simulink model "DCMotor_Para_Est_2021b"  (R2021b)
settings: Solver=VariableStepAuto  StartTime=0.0  StopTime=10.0  RelTol=1e-3
libraries: arduinolib x2, arduinosensorlib x1
settings Model: Creator=LabPC  LastModifiedBy=LabPC
settings DebuggingCC: UnconnectedInputMsg=none  UnconnectedOutputMsg=none  UnconnectedLineMsg=none
settings RTWCC: DLArmComputeVersion=20.02.1

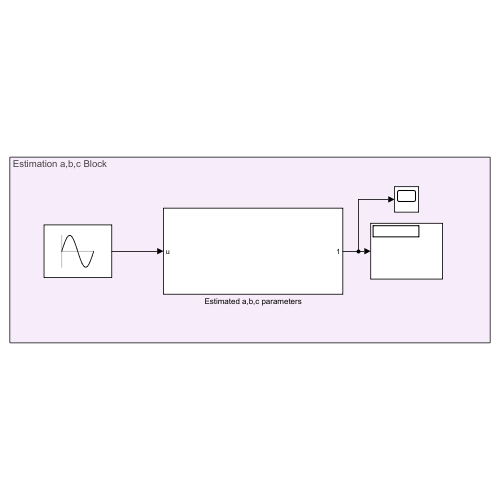
[thumbnail: Simulink's stored preview of the top-level diagram]
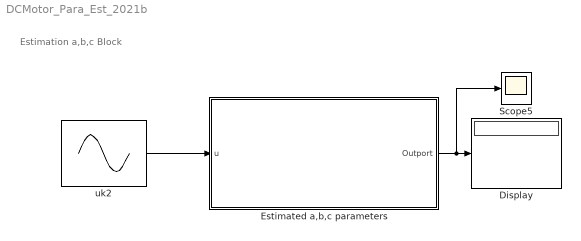
== system DCMotor_Para_Est_2021b ==
  note: Estimation a,b,c Block
  Display : Display
  Estimated a,b,c parameters : Subsystem
  Scope5 : Scope
  uk2 : Sin  Amplitude=12  Frequency=2*pi*1.2  SampleTime=0
  wires:
  Estimated a,b,c parameters/1(Outport) -> Scope5/1, Display/1
  uk2/1 -> Estimated a,b,c parameters/1(u)

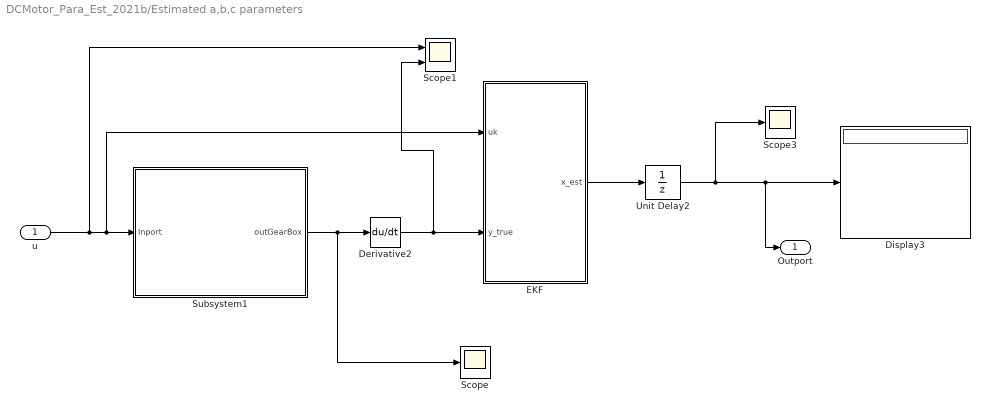
== system DCMotor_Para_Est_2021b/Estimated a,b,c parameters ==
  u : Inport
  Derivative2 : Derivative
  Display3 : Display
  EKF : MATLAB Function  TreatAsAtomicUnit=on
  Scope : Scope
  Scope1 : Scope  NumInputPorts=2
  Scope3 : Scope
  Subsystem1 : Subsystem
  Unit Delay2 : UnitDelay  InitialCondition=[0;0;0;0]  SampleTime=-1  HasFrameUpgradeWarning=on
  Outport : Outport
  wires:
  Derivative2/1 -> Scope1/2, EKF/2(y_true)
  Unit Delay2/1 -> Outport/1, Display3/1, Scope3/1
  EKF/1(x_est) -> Unit Delay2/1
  Subsystem1/1(outGearBox) -> Scope/1, Derivative2/1
  u/1 -> Scope1/1, Subsystem1/1(Inport), EKF/1(uk)

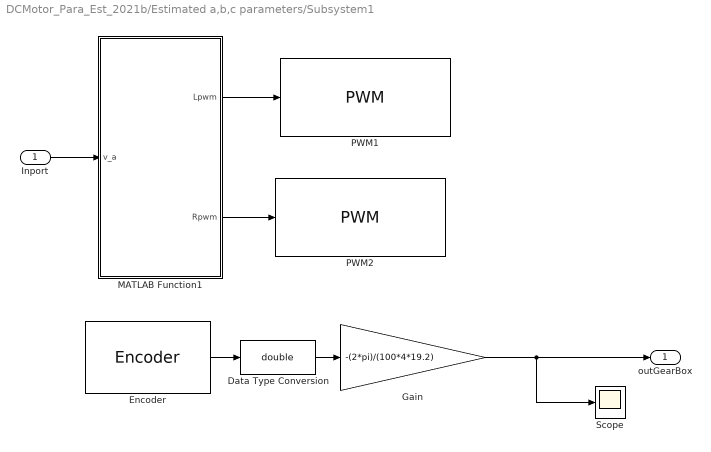
== system DCMotor_Para_Est_2021b/Estimated a,b,c parameters/Subsystem1 ==
  Inport : Inport
  Data Type Conversion : DataTypeConversion  OutDataTypeStr=double
  Encoder : arduinosensorlib/Encoder  InputA=2  InputB=3  Mode=No reset  SampleTime=-1
      settings: SourceProductBaseCode=ARDUINO
  Gain : Gain  Gain=-(2*pi)/(100*4*19.2)
  MATLAB Function1 : MATLAB Function  TreatAsAtomicUnit=on
  PWM1 : arduinolib/PWM  pinNumber=6  frequencyType=Default  desiredFrequency=490.2  achievableFrequency=490.2
  PWM2 : arduinolib/PWM  pinNumber=7  frequencyType=Default  desiredFrequency=490.2  achievableFrequency=490.2
  Scope : Scope
  outGearBox : Outport
  wires:
  Gain/1 -> Scope/1, outGearBox/1
  Encoder/1 -> Data Type Conversion/1
  Data Type Conversion/1 -> Gain/1
  MATLAB Function1/1(Lpwm) -> PWM1/1
  MATLAB Function1/2(Rpwm) -> PWM2/1
  Inport/1 -> MATLAB Function1/1(v_a)

== matlab function DCMotor_Para_Est_2021b/Estimated a,b,c parameters/Subsystem1/MATLAB Function1 ==
  data: v_a input; Lpwm output; Rpwm output
function [Lpwm,Rpwm] = fcn(v_a)

vmax = 22.9;
pwm_cal = v_a*254/vmax;

if pwm_cal > 0
    Lpwm = 0;
    Rpwm = pwm_cal;
elseif pwm_cal < 0
    Lpwm = abs(pwm_cal);
    Rpwm = 0;
else
    Lpwm = 0;
    Rpwm = 0;
end

== matlab function DCMotor_Para_Est_2021b/Estimated a,b,c parameters/EKF ==
  settings: updateMethod=DISCRETE
  data: uk input; y_true input; x_est output
function x_est = fcn(uk,y_true)
Ts=0.01;
persistent x_est_p P Qd_est R_est Qc_est;
if isempty(x_est_p)
          
          x_est_p=[2;16;3.5;2];
          P=2*eye(4);
         Qc_est=1e-3*diag([10,10,10,1]);
          Qd_est=Qc_est*Ts;
          R_est=0.02;
end
c=[1 0 0 0];D=0;Ck=c;Dk=D;
%Comput Kalman Gain and update predicted value
Wk=P*Ck'/(Ck*P*Ck'+R_est);
y_est=Ck*x_est_p+Dk*uk;
x=x_est_p+Wk.*(y_true-y_est);
%Compute prediction at next time step
x_est=x+Ts*[-x(2)*x(1)+uk*x(3)-x(4)*sign(x(1));0;0;0];
%Update error covariance matrices
P=P-Wk*Ck*P;
%Define Ak
Ak=eye(4)+Ts*[-x(2) -x(1) uk -sign(x(1));0 0 0 0;0 0 0 0;0 0 0 0];
P=Ak*P*Ak'+Qd_est;
x_est_p=x_est;
